simulink subsystem "Acceleration_in_Geodetic_Frame"  (R2022a)
settings: Solver=VariableStepAuto  StartTime=0.0  StopTime=10.0  RelTol=1e-3
libraries: matrix_library x1
settings Model: Creator=Andrew Radulovich  LastModifiedBy=Andrew Radulovich

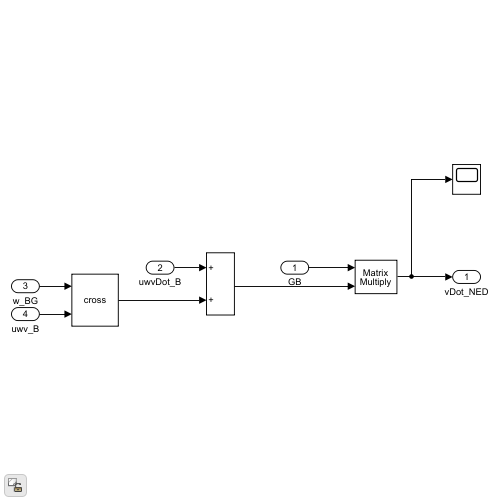
[thumbnail: Simulink's stored preview of the top-level diagram]
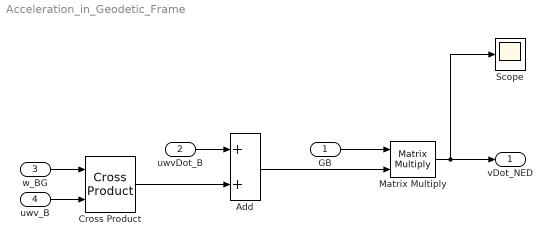
== system Acceleration_in_Geodetic_Frame ==
  GB : Inport
  uwvDot_B : Inport  Port=2
  w_BG : Inport  Port=3
  uwv_B : Inport  Port=4
  Add : Sum
  Cross Product : matrix_library/Cross Product
      settings: SourceProductBaseCode=SL
  Matrix Multiply : Product  Multiplication=Matrix(*)
  Scope : Scope
  vDot_NED : Outport
  wires:
  GB/1 -> Matrix Multiply/1
  uwvDot_B/1 -> Add/1
  uwv_B/1 -> Cross Product/2
  w_BG/1 -> Cross Product/1
  Cross Product/1 -> Add/2
  Add/1 -> Matrix Multiply/2
  Matrix Multiply/1 -> vDot_NED/1, Scope/1
